simulink model "CONTROLADORpidDIGITAL"  (R2023a)
settings: Solver=VariableStepAuto  StartTime=0.0  StopTime=3  RelTol=1e-3
undefined symbols (not defined in the file): kd, ki, kp
settings Model: Creator=a2150336  LastModifiedBy=a2150336

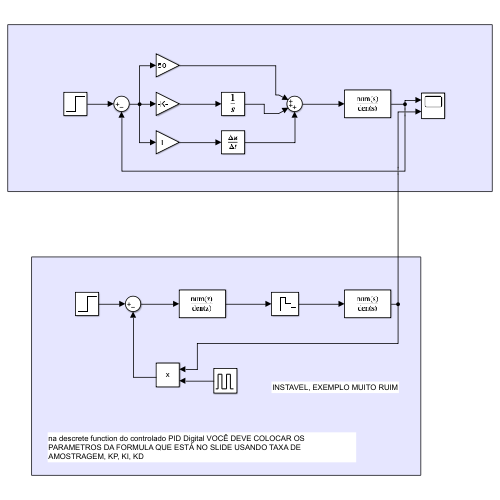
[thumbnail: Simulink's stored preview of the top-level diagram]
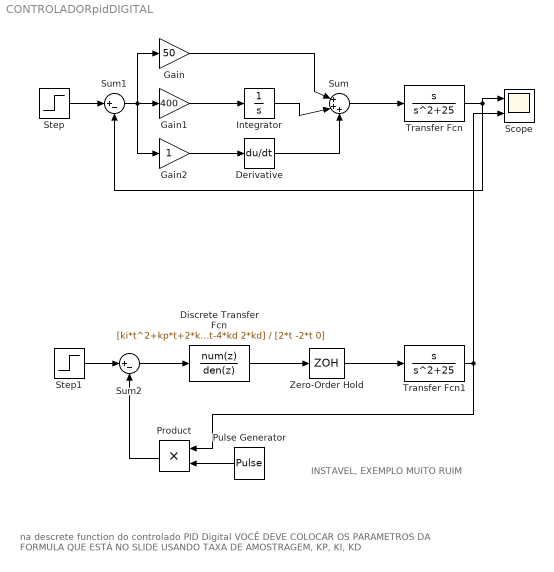
== system CONTROLADORpidDIGITAL ==
  note: INSTAVEL, EXEMPLO MUITO RUIM
  note: na descrete function do controlado PID Digital VOCÊ DEVE COLOCAR OS PARAMETROS DA FORMULA QUE ESTÁ NO SLIDE USANDO TAXA DE AMOSTRAGEM, KP, KI, KD
  Derivative : Derivative
  Discrete Transfer Fcn : DiscreteTransferFcn  Numerator=[ki*t^2+kp*t+2*kd ki*t^2-2*kp*t-4*kd 2*kd]  Denominator=[2*t -2*t 0]
  Gain : Gain  Gain=50
  Gain1 : Gain  Gain=400
  Gain2 : Gain
  Integrator : Integrator
  Product : Product
  Pulse Generator : DiscretePulseGenerator  PulseType=Time based  Period=10  PulseWidth=5
  Scope : Scope  NumInputPorts=2
  Step : Step  SampleTime=0
  Step1 : Step  SampleTime=0
  Sum : Sum  Inputs=|+++
  Sum1 : Sum  Inputs=|+-
  Sum2 : Sum  Inputs=|+-
  Transfer Fcn : TransferFcn  Numerator=[1 0]  Denominator=[1 0 25]
  Transfer Fcn1 : TransferFcn  Numerator=[1 0]  Denominator=[1 0 25]
  Zero-Order Hold : ZeroOrderHold  SampleTime=-1
  wires:
  Gain1/1 -> Integrator/1
  Integrator/1 -> Sum/2
  Derivative/1 -> Sum/3
  Gain/1 -> Sum/1
  Sum/1 -> Transfer Fcn/1
  Transfer Fcn/1 -> Sum1/2, Scope/1
  Sum1/1 -> Gain2/1, Gain/1, Gain1/1
  Step/1 -> Sum1/1
  Gain2/1 -> Derivative/1
  Step1/1 -> Sum2/1
  Sum2/1 -> Discrete Transfer Fcn/1
  Pulse Generator/1 -> Product/2
  Zero-Order Hold/1 -> Transfer Fcn1/1
  Discrete Transfer Fcn/1 -> Zero-Order Hold/1
  Transfer Fcn1/1 -> Scope/2, Product/1
  Product/1 -> Sum2/2
